simulink model "WZ_CAE_4_1"  (R2023b)
settings: Solver=VariableStepAuto  StartTime=0.0  StopTime=200  RelTol=1e-3
libraries: simulink x1
settings Model: Creator=user  LastModifiedBy=Wojciech Zub
settings SolverCC: AlgebraicLoopSolver=TrustRegion
settings DebuggingCC: UnconnectedInputMsg=warning  UnconnectedOutputMsg=warning  UnconnectedLineMsg=warning
settings ModelReferenceCC: EnableRefExpFcnMdlSchedulingChecks=on

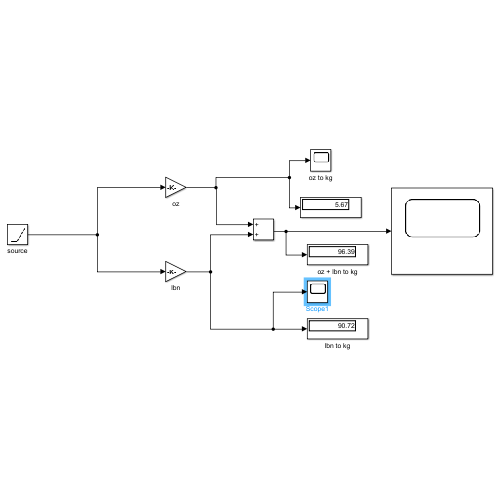
[thumbnail: Simulink's stored preview of the top-level diagram]
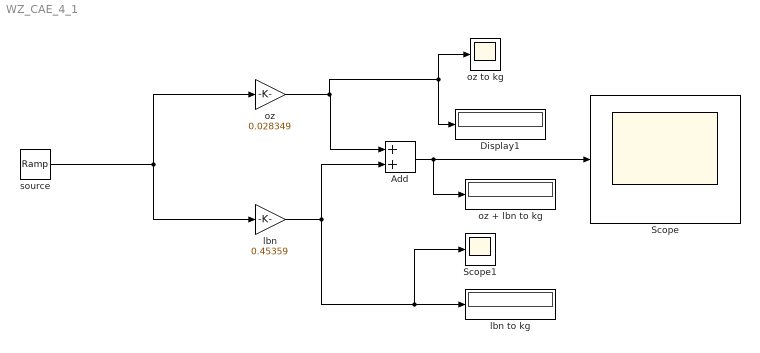
== system WZ_CAE_4_1 ==
  Add : Sum
  Display1 : Display
  Scope : Scope
  Scope1 : Scope
  lbn : Gain  Gain=0.45359
  lbn to kg : Display
  oz : Gain  Gain=0.028349
  oz + lbn to kg : Display
  oz to kg : Scope
  source : simulink/Sources/Ramp  slope=1  start=0  InitialOutput=0
  wires:
  Add/1 -> oz + lbn to kg/1, Scope/1
  oz/1 -> Display1/1, oz to kg/1, Add/1
  source/1 -> lbn/1, oz/1
  lbn/1 -> Add/2, Scope1/1, lbn to kg/1
